simulink model "filter_test"  (R2023b)
settings: Solver=VariableStepAuto  StartTime=0.0  StopTime=Tend  RelTol=1e-3
values from neighbouring files (symbols this model uses):
  meas_pole = 10    [main_motor_noise_analysis.m]
  Ts_slk = 0.01    [main_motor_noise_analysis.m]
settings Model: Creator=teoma  LastModifiedBy=teoma

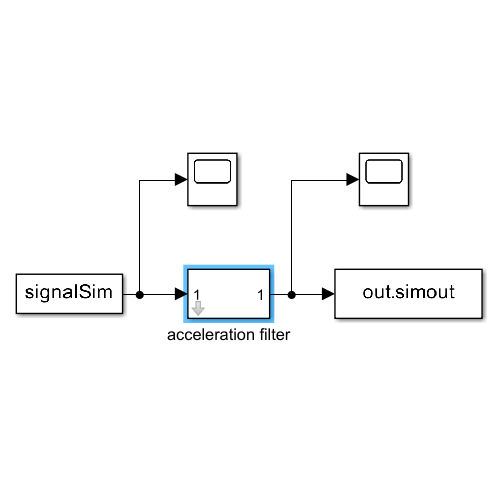
[thumbnail: Simulink's stored preview of the top-level diagram]
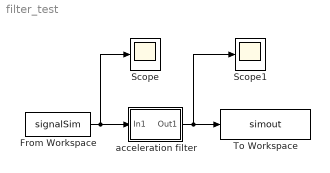
== system filter_test ==
  From Workspace : FromWorkspace  VariableName=signalSim  SampleTime=Ts_slk
  Scope : Scope
  Scope1 : Scope
  To Workspace : ToWorkspace  VariableName=simout  SampleTime=-1
  acceleration filter : Subsystem  mask{p=meas_pole}
      mask prompts: p "pole (p)"
  wires:
  From Workspace/1 -> Scope/1, acceleration filter/1(In1)
  acceleration filter/1(Out1) -> Scope1/1, To Workspace/1

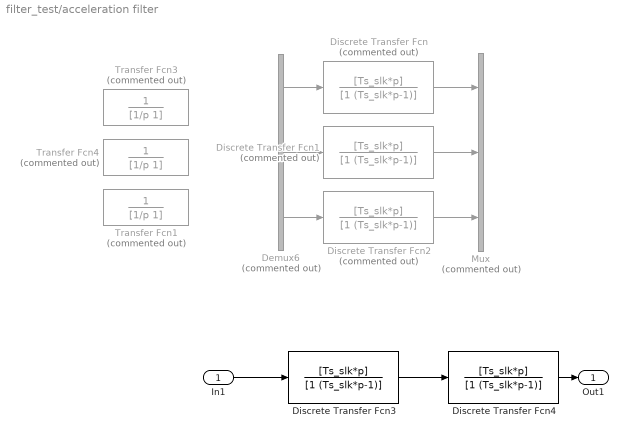
== system filter_test/acceleration filter ==
  In1 : Inport
  Demux6 : Demux  Commented=on  Outputs=3
  Discrete Transfer Fcn : DiscreteTransferFcn  Commented=on  Numerator=[Ts_slk*p]  Denominator=[1 (Ts_slk*p-1)]
  Discrete Transfer Fcn1 : DiscreteTransferFcn  Commented=on  Numerator=[Ts_slk*p]  Denominator=[1 (Ts_slk*p-1)]
  Discrete Transfer Fcn2 : DiscreteTransferFcn  Commented=on  Numerator=[Ts_slk*p]  Denominator=[1 (Ts_slk*p-1)]
  Discrete Transfer Fcn3 : DiscreteTransferFcn  Numerator=[Ts_slk*p]  Denominator=[1 (Ts_slk*p-1)]
  Discrete Transfer Fcn4 : DiscreteTransferFcn  Numerator=[Ts_slk*p]  Denominator=[1 (Ts_slk*p-1)]
  Mux : Mux  Commented=on  Inputs=3
  Transfer Fcn1 : TransferFcn  Commented=on  Denominator=[1/p 1]
  Transfer Fcn3 : TransferFcn  Commented=on  Denominator=[1/p 1]
  Transfer Fcn4 : TransferFcn  Commented=on  Denominator=[1/p 1]
  Out1 : Outport
  wires:
  Demux6/1 -> Discrete Transfer Fcn/1
  Demux6/2 -> Discrete Transfer Fcn1/1
  Discrete Transfer Fcn1/1 -> Mux/2
  Discrete Transfer Fcn2/1 -> Mux/3
  Demux6/3 -> Discrete Transfer Fcn2/1
  Discrete Transfer Fcn/1 -> Mux/1
  In1/1 -> Discrete Transfer Fcn3/1
  Discrete Transfer Fcn3/1 -> Discrete Transfer Fcn4/1
  Discrete Transfer Fcn4/1 -> Out1/1
